simulink model "Basic_3ph"  (R2025a)
settings: Solver=VariableStepAuto  StartTime=0.0  StopTime=0.5  MaxStep=T_s  RelTol=1e-3
values from neighbouring files (symbols this model uses):
  Cdc = 500e-6    (= 0.0005)    [simulik_parameter_setter_inverter.m]
  f_e = 500    [simulik_parameter_setter_inverter.m]
  L_ph = 0.25e-3    (= 0.00025)    [simulik_parameter_setter_inverter.m]
  R_ph = 0.8e-3    (= 0.0008)    [ISCAD_Coupled_Model_3ph.m]
  T_s = 1/(20*f_sw)    [PowerElectronics_Analytical.m]    (also in simulik_parameter_setter_inverter.m = 2e-06)
  Td = 2e-6    (= 2e-06)    [PowerElectronics_Analytical.m]    (also in simulik_parameter_setter_inverter.m)
  Vdc = 48    [PowerElectronics_Analytical.m]    (also in simulik_parameter_setter_inverter.m)
undefined symbols (not defined in the file or in its folder): m
libraries: nesl_utility x14, fl_lib x9, ee_lib x6, eePwmGeneratorTwoLevel x1, spsRMSLib x1, spsThreePhaseSineGeneratorLib x1
settings Model: Creator=ossia  LastModifiedBy=ossia

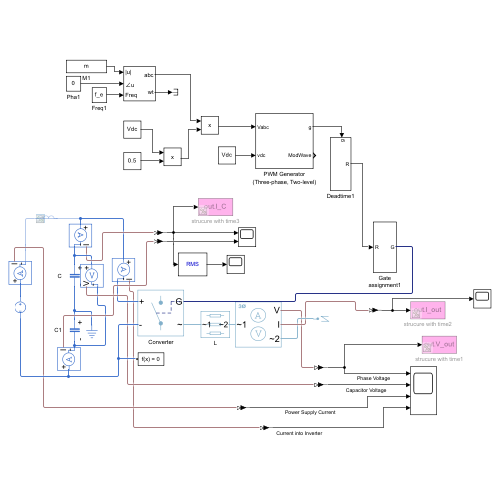
[thumbnail: Simulink's stored preview of the top-level diagram]
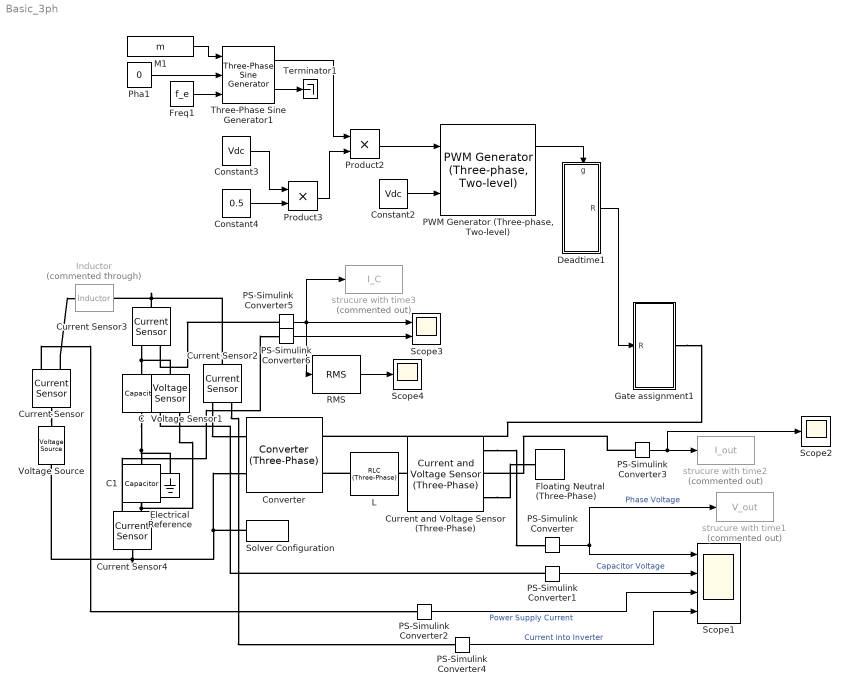
== system Basic_3ph ==
  C : fl_lib/Electrical/Electrical Elements/Capacitor  c=3*Cdc/2 uF  r=1e-4 Ohm  g=0 1/Ohm  i_specify=off  i_priority=High  i=0 A  i_nominal_specify=off  i_nominal_value=1  i_nominal_unit=A  v_specify=off  v_priority=None  v=Vdc/2 V  v_nominal_specify=off  v_nominal_value=1  v_nominal_unit=V  vc_specify=on  vc_priority=High  vc=Vdc/2 V  vc_nominal_specify=off  vc_nominal_value=1  vc_nominal_unit=V
  C1 : fl_lib/Electrical/Electrical Elements/Capacitor  c=3*Cdc/2 uF  r=1e-4 Ohm  g=0 1/Ohm  i_specify=off  i_priority=High  i=0 A  i_nominal_specify=off  i_nominal_value=1  i_nominal_unit=A  v_specify=off  v_priority=None  v=46 V  v_nominal_specify=off  v_nominal_value=1  v_nominal_unit=V  vc_specify=on  vc_priority=High  vc=Vdc/2 V  vc_nominal_specify=off  vc_nominal_value=1  vc_nominal_unit=V
  Constant2 : Constant  Value=Vdc
  Constant3 : Constant  Value=Vdc
  Constant4 : Constant  Value=0.5
  Converter : ee_lib/Semiconductors & Converters/Converters/Converter (Three-Phase)  port_option=ee.enum.threePhasePort.composite  fidelity_option=ee.enum.converters.fidelity.equivalent_pwm  device_type=ee.enum.converters.switchingdevice.mosfet  showThermalPort=false  K=0  Vth=0.5 V  Vgt=0.5 V  Vgt_off=0.1 V  Ih=1 A  Vf=0.6 V  Ron=0.002 Ohm  Rds=0.002 Ohm  Goff=1e-6 S  Eon_scalar=22.86e-3 J  Eoff_scalar=17.14e-3 J  Eoff_natural_commutation=10e-3 J  Voff=300 V  Iout_scalar=600 A  onCurrentMeasDelay=0 s  useCurrentFromPreviousCycle=false  useVoltageFromPreviousCycle=false  diode_param=2  diode_Vf=0.8 V  diode_Ron=0.001 Ohm  diode_Goff=1e-5 S  diode_C=5e-8 F  diode_iRM=-235 A  diode_iF=300 A  diode_idot=-50 A/us  diode_trr_param=1  diode_trr_factor=3  diode_trr=15 us  diode_Qrr=1.5e+3 s*uA  diode_rec_loss_model=ee.enum.diode.reverseRecoveryModel.fixed  diode_ErecVal=0 J  diode_scaleWithIandV=false  diode_ErecMat=zeros(2, 3) J  diode_TjrecVec=[298.15, 398.15] K  diode_IfrecVec=[.1, 1, 10] A  diode_IrecVal=10 A  diode_VrecVal=10 V  diode_tFilter=1 / 1000 / 100 s  thermal_network_parameterization=ee.enum.thermalNetworkTopology.external  Rth=[.08, .5] K/W  Rth_Cauer=[.08, .1, .5] K/W  Rth_Foster=[.08, .14, .22, .16] K/W  thermal_mass_parameterization=ee.enum.thermalNetwork.timeconstant  thermal_mass=[.01, .5] J/K  thermal_mass_Cauer=[.01, .1, .5] J/K  thermal_mass_Foster=[.001, .005, .05, .5] J/K  thermal_time_constant=[.001, .2] s  thermal_time_constant_Cauer=[.001, .1, .2] s  thermal_time_constant_Foster=[7e-05, .0007, .01, .08] s  thermal_mass_initial_temperatures=[25, 25] degC  thermal_mass_initial_temperatures_Cauer=[25, 25, 25] degC  junction_thermal_mass=0.01 J/K  Tvec_initial_Foster=[25, 25, 25, 25] degC  snubber_type=ee.enum.converters.snubber.exclude  Cs=1e-7 F  Rs=0.1 Ohm  Vce_loss=[0, 150, 300] V
  Current Sensor{,2..4} (4 alike) : fl_lib/Electrical/Electrical Sensors/Current Sensor
  Current and Voltage Sensor (Three-Phase) : ee_lib/Sensors & Transducers/Current and Voltage Sensor (Three-Phase)  vMeasurementType=ee.enum.vmeasurement.lg  outputUnit=ee.enum.unit.si  SRated=100e6 A*V  VRated=24e3 V  I_specify=off  I_priority=None  I=[0, 0, 0] A  I_nominal_specify=off  I_nominal_value=1  I_nominal_unit=A  V_specify=off  V_priority=None  V=[0, 0, 0] V  V_nominal_specify=off  V_nominal_value=1  V_nominal_unit=V
      settings: InternalSimscapePortConfiguration="{\"Bottom\":[],\"Left\":[{\"id\":\"N1\",\"label\":\"~1\",\"type\":\"foundation.electrical.three_phase\"}],\"Right\":[{\"id\":\"V_output\",\"label\":\"V\",\"type\":\"output\"},{\"id\":\"I_output\",\"label\":\"I\",\"type\":\"output\"},{\"id\":\"N2\",\"label\":\"~2\",\"type\":\"foundation.electrical.three_phase\"}],\"Top\":[]}"
  Deadtime1 : Subsystem
      settings: PortSchema="{\"entries\":[{\"content\":{\"sides\":[{\"content\":{\"connectorIds\":[\"Out1\"]},\"type\":\"ConnectorPlacement.EquallySpacedRectSide\",\"uuid\":\"80ef36b9-f465-4fcc-93a9-9d6eab044ae8\"},{\"content\":{\"side\":\"RIGHT\"},\"type\":\"ConnectorPlacement.EquallySpacedRectSide\",\"uuid\":\"10827d79-0026-467d-af8f-e653363972a6\"},{\"content\":{\"connectorIds\":[\"In1\"],\"side\":\"TOP\"},\"type\":\"ConnectorPlacement.EquallySpacedRectSide\",\"uuid\":\"d9163dac-283f-4784-a2ff-48ce53974a1a\"}]},\"type\":\"ConnectorPlacement.EquallySpacedConnector\",\"uuid\":\"7e643ad6-bdf3-49e0-97a6-0ece4f3a3f1f\"}],\"packageUris\":[\"http://schema.mathworks.com/mf0/Connector/R2020b\"],\"version\":\"1.0\"}"
  Electrical Reference : fl_lib/Electrical/Electrical Elements/Electrical Reference
  Floating Neutral (Three-Phase) : ee_lib/Connectors & References/Floating Neutral (Three-Phase)  G_parasitic=1e-12 1/Ohm
      settings: InternalSimscapePortConfiguration="{\"Bottom\":[],\"Left\":[{\"id\":\"N\",\"label\":\"~\",\"type\":\"foundation.electrical.three_phase\"}],\"Right\":[],\"Top\":[]}"
  Freq1 : Constant  Value=f_e
  Gate assignment1 : Subsystem
  Inductor : fl_lib/Electrical/Electrical Elements/Inductor  Commented=through  l=3*L_ph H  r=2e-3 Ohm  g=1e-9 1/Ohm  i_specify=off  i_priority=None  i=2 A  i_nominal_specify=off  i_nominal_value=1  i_nominal_unit=A  v_specify=off  v_priority=None  v=0 V  v_nominal_specify=off  v_nominal_value=1  v_nominal_unit=V  i_L_specify=off  i_L_priority=High  i_L=2 A  i_L_nominal_specify=off  i_L_nominal_value=1  i_L_nominal_unit=A
  L : ee_lib/Passive/RLC Assemblies/RLC (Three-Phase)  port_option=ee.enum.threePhasePort.composite  component_structure=4  R=R_ph Ohm  L=L_ph H  C=1e-6 F  R_parasitic=1e-6 Ohm  G_parasitic=1e-6 1/Ohm  IL_specify=on  IL_priority=High  IL=[ -14 7 7 ] A  IL_nominal_specify=off  IL_nominal_value=1  IL_nominal_unit=A  VC_specify=on  VC_priority=High  VC=[ 0 0 0 ] V  VC_nominal_specify=off  VC_nominal_value=1  VC_nominal_unit=V
      settings: InternalSimscapePortConfiguration="{\"Bottom\":[],\"Left\":[{\"id\":\"N1\",\"label\":\"~1\",\"type\":\"foundation.electrical.three_phase\"}],\"Right\":[{\"id\":\"N2\",\"label\":\"~2\",\"type\":\"foundation.electrical.three_phase\"}],\"Top\":[]}"
  M1 : Constant  Value=m
  PS-Simulink Converter{,1..6} (7 alike) : nesl_utility/PS-Simulink Converter  PhysicalDomain=network_engine_domain  SubClassName=ps_output  LeftPortType=input  RightPortType=output  PseudoPeriodic=off  Frequencies=[]  VectorFormat=inherit  Unit=inherit  AffineConversion=off
  "PWM Generator (Three-phase, Two-level)" : eePwmGeneratorTwoLevel/PWM Generator (Three-phase, Two-level)  PWMMode=Continuous PWM (CPWM)  CPWMMode=SPWM: sinusoidal PWM  DPWMMode=30 DPWM: 30 degree discontinuous PWM  fsw=f_sw  Ts=T_s
      settings: SamplingMode=Asymmetric
      settings: LibrarySourceBlock=|
      | ee_sl_lib/Pulse Width
      | Modulation/PWM Generator
      | (Three-phase, Two-level)
  Pha1 : Constant  Value=0
  Product2 : Product
  Product3 : Product
  RMS : spsRMSLib/RMS  TrueRMS=on  Freq=25  RMSInit=0  Ts=T_s
  Scope1 : Scope  NumInputPorts=4
      settings: ActiveDisplayYMinimum=-29.00001636217473  ActiveDisplayYMaximum=21.000035118664378
  Scope2 : Scope
      settings: ActiveDisplayYMinimum=-1023.5079890337755  ActiveDisplayYMaximum=992.075721007424  DataLoggingVariableName=ScopeData2
  Scope3 : Scope  NumInputPorts=2
      settings: ActiveDisplayYMinimum=-298.34389890666739  ActiveDisplayYMaximum=287.62683048751734  DataLoggingVariableName=ScopeData3
  Scope4 : Scope
      settings: ActiveDisplayYMinimum=-372.34194  ActiveDisplayYMaximum=490.06934
  Solver Configuration : nesl_utility/Solver Configuration  PhysicalDomain=network_engine_domain  SubClassName=solver  LeftPortType=input  RightPortType=generic  Tones=[]  Harmonics=[]  SimulateNoise=off  Profile=off  UseLocalSampling=off  EnableSwitchedLinearOptims=on  FrequencyDomain=off  UseCCode=off  RelTol=0.001  AbsTol=1e-06  MinStep=1e-09  ToWorkspace=off  RevertToSquareIcSolve=off  NumHomotopyIterations=100  PhasorMode=off  PhasorModeNumHarmonics=1  ConsistencySolver=NEWTON_FTOL  IndexReductionMethod=DerivativeReplacement  DoDC=off  ResidualTolerance=1e-09  ConsistencyTolSource=GLOBAL  ConsistencyAbsTol=0.001  ConsistencyRelTol=0.001  ConsistencyTolFactor=0.001  UseLocalSolver=off  LocalSolverChoice=NE_BACKWARD_EULER_ADVANCER  ResolveIndetEquations=on  FunctionEvalNumThread=1  LocalSolverSampleTime=1e-5  DoFixedCost=off  MaxNonlinIter=5  MaxModeIter=2  ComputeImpulses=off  ImpulseIterations=2  LinearAlgebra=Sparse  LinearAlgebraNumThread=0  EquationFormulation=NE_TIME_EF  DelaysMemoryBudget=1024  AutomaticFiltering=on  FilteringTimeConstant=0.001  PartitionStorageMethod=AS_NEEDED  PartitionMemoryBudget=1024  PartitionMethod=FAST  MultibodyUseLocalSolver=off  MultibodyLocalSolverChoice=ODE1  MultibodyLocalSolverSampleTime=0.001
  Terminator1 : Terminator
  Three-Phase Sine Generator1 : spsThreePhaseSineGeneratorLib/Three-Phase Sine Generator  Ts=T_s
      settings: LibrarySourceBlock=|
      | sps_lib/Sources/Signal Generator Sources/Three-Phase
      | Sine Generator
  Voltage Sensor1 : fl_lib/Electrical/Electrical Sensors/Voltage Sensor
  Voltage Source : ee_lib/Sources/Voltage Source  dc_voltage=Vdc V  ac_voltage=0 V  ac_shift=0 rad  ac_frequency=0 Hz  noise_mode=ee.enum.sources.noise.Disabled  PSD=0 V^2/Hz  sample_time=1e-3 s  repeatability=ee.enum.sources.repeatability.NotRepeatable  user_seed=0  auto_seed=3890346746  i_specify=off  i_priority=None  i=0 A  i_nominal_specify=off  i_nominal_value=1  i_nominal_unit=A  v_specify=off  v_priority=None  v=0 V  v_nominal_specify=off  v_nominal_value=1  v_nominal_unit=V
  strucure with time1 : ToWorkspace  Commented=on  VariableName=V_out  SaveFormat=Structure With Time  SampleTime=T_s
  strucure with time2 : ToWorkspace  Commented=on  VariableName=I_out  SaveFormat=Structure With Time  SampleTime=T_s
  strucure with time3 : ToWorkspace  Commented=on  VariableName=I_C  SaveFormat=Structure With Time  SampleTime=T_s
  wires:
  PS-Simulink Converter/1 -> strucure with time1/1, Scope1/1  "Phase Voltage"
  Constant4/1 -> Product3/2
  Three-Phase Sine Generator1/1 -> Product2/1
  Freq1/1 -> Three-Phase Sine Generator1/3
  PS-Simulink Converter1/1 -> Scope1/2  "Capacitor Voltage"
  Deadtime1/1(R) -> Gate assignment1/1(R)
  Pha1/1 -> Three-Phase Sine Generator1/2
  PS-Simulink Converter6/1 -> Scope3/2
  Three-Phase Sine Generator1/2 -> Terminator1/1
  Constant2/1 -> "PWM Generator (Three-phase, Two-level)"/2
  Product2/1 -> "PWM Generator (Three-phase, Two-level)"/1
  "PWM Generator (Three-phase, Two-level)"/1 -> Deadtime1/1(g)
  PS-Simulink Converter2/1 -> Scope1/3  "Power Supply Current"
  PS-Simulink Converter3/1 -> Scope2/1, strucure with time2/1
  Product3/1 -> Product2/2
  PS-Simulink Converter5/1 -> strucure with time3/1, RMS/1, Scope3/1
  RMS/1 -> Scope4/1
  Constant3/1 -> Product3/1
  PS-Simulink Converter4/1 -> Scope1/4  "Current into Inverter"
  M1/1 -> Three-Phase Sine Generator1/1
  connections:
  Converter/RConn2 -- Solver Configuration/RConn1 -- Current Sensor4/LConn1 -- Voltage Source/RConn1
  C1/LConn1 -- C/RConn1 -- Electrical Reference/LConn1
  C/LConn1 -- Voltage Sensor1/LConn1 -- Current Sensor3/RConn2
  Current Sensor3/LConn1 -- Current Sensor2/LConn1 -- Inductor/RConn1
  PS-Simulink Converter5/LConn1 -- Current Sensor3/RConn1
  Current Sensor/RConn2 -- Inductor/LConn1
  PS-Simulink Converter1/LConn1 -- Voltage Sensor1/RConn1
  Current Sensor/RConn1 -- PS-Simulink Converter2/LConn1
  PS-Simulink Converter3/LConn1 -- Current and Voltage Sensor (Three-Phase)/RConn2
  Current Sensor4/RConn1 -- PS-Simulink Converter6/LConn1
  Current Sensor2/RConn1 -- PS-Simulink Converter4/LConn1
  Gate assignment1/RConn1 -- Converter/LConn1
  Current Sensor4/RConn2 -- Voltage Sensor1/RConn2 -- C1/RConn1
  Current Sensor2/RConn2 -- Converter/RConn1
  Current Sensor/LConn1 -- Voltage Source/LConn1
  Current and Voltage Sensor (Three-Phase)/RConn1 -- PS-Simulink Converter/LConn1
  L/LConn1 -- Converter/LConn2
  Current and Voltage Sensor (Three-Phase)/LConn1 -- L/RConn1
  Current and Voltage Sensor (Three-Phase)/RConn3 -- Floating Neutral (Three-Phase)/LConn1

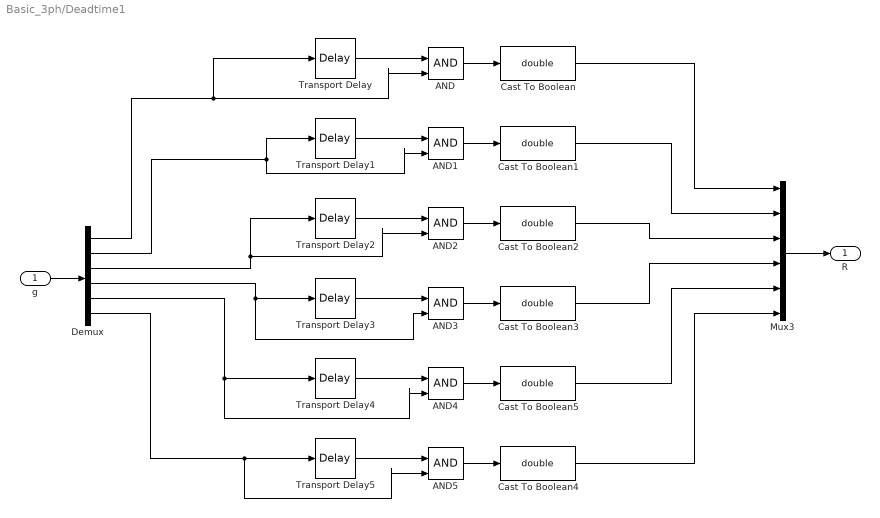
== system Basic_3ph/Deadtime1 ==
  g : Inport
  AND{,1..5} (6 alike) : Logic  IconShape=distinctive  AllPortsSameDT=off  OutDataTypeStr=boolean
  Cast To Boolean{,1..5} (6 alike) : DataTypeConversion  OutDataTypeStr=double  SaturateOnIntegerOverflow=off  RndMeth=Floor
  Demux : Demux  Outputs=6
  Mux3 : Mux  Inputs=6
  Transport Delay{,1..5} (6 alike) : TransportDelay  DelayTime=Td
  R : Outport
  wires:
  g/1 -> Demux/1
  Transport Delay/1 -> AND/1
  Demux/1 -> Transport Delay/1, AND/2
  AND/1 -> Cast To Boolean/1
  Demux/2 -> Transport Delay1/1, AND1/2
  Transport Delay1/1 -> AND1/1
  Transport Delay2/1 -> AND2/1
  AND2/1 -> Cast To Boolean2/1
  Demux/3 -> Transport Delay2/1, AND2/2
  Demux/4 -> AND3/2, Transport Delay3/1
  Transport Delay3/1 -> AND3/1
  Demux/5 -> AND4/2, Transport Delay4/1
  Transport Delay4/1 -> AND4/1
  AND4/1 -> Cast To Boolean5/1
  Demux/6 -> AND5/2, Transport Delay5/1
  Transport Delay5/1 -> AND5/1
  AND1/1 -> Cast To Boolean1/1
  AND3/1 -> Cast To Boolean3/1
  AND5/1 -> Cast To Boolean4/1
  Cast To Boolean/1 -> Mux3/1
  Cast To Boolean1/1 -> Mux3/2
  Cast To Boolean2/1 -> Mux3/3
  Cast To Boolean3/1 -> Mux3/4
  Cast To Boolean5/1 -> Mux3/5
  Cast To Boolean4/1 -> Mux3/6
  Mux3/1 -> R/1

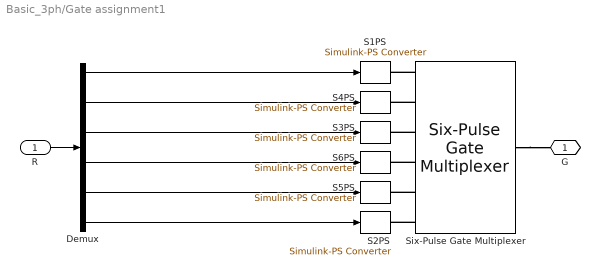
== system Basic_3ph/Gate assignment1 ==
  R : Inport
  Demux : Demux  Outputs=6
  S1PS : nesl_utility/Simulink-PS Converter  PhysicalDomain=network_engine_domain  SubClassName=ps_input  LeftPortType=input  RightPortType=output  PseudoPeriodic=off  Frequencies=[]  NoiseDistribution=none  NoiseParameters=[]  Unit=1  AffineConversion=off  FilteringAndDerivatives=zero  SimscapeFilterOrder=1  InputFilterTimeConstant=.001  UdotUserProvided=1
  S2PS : nesl_utility/Simulink-PS Converter  PhysicalDomain=network_engine_domain  SubClassName=ps_input  LeftPortType=input  RightPortType=output  PseudoPeriodic=off  Frequencies=[]  NoiseDistribution=none  NoiseParameters=[]  Unit=1  AffineConversion=off  FilteringAndDerivatives=zero  SimscapeFilterOrder=1  InputFilterTimeConstant=.001  UdotUserProvided=[]
  S3PS : nesl_utility/Simulink-PS Converter  PhysicalDomain=network_engine_domain  SubClassName=ps_input  LeftPortType=input  RightPortType=output  PseudoPeriodic=off  Frequencies=[]  NoiseDistribution=none  NoiseParameters=[]  Unit=1  AffineConversion=off  FilteringAndDerivatives=zero  SimscapeFilterOrder=1  InputFilterTimeConstant=.001  UdotUserProvided=[]
  S4PS : nesl_utility/Simulink-PS Converter  PhysicalDomain=network_engine_domain  SubClassName=ps_input  LeftPortType=input  RightPortType=output  PseudoPeriodic=off  Frequencies=[]  NoiseDistribution=none  NoiseParameters=[]  Unit=1  AffineConversion=off  FilteringAndDerivatives=zero  SimscapeFilterOrder=1  InputFilterTimeConstant=.001  UdotUserProvided=[]
  S5PS : nesl_utility/Simulink-PS Converter  PhysicalDomain=network_engine_domain  SubClassName=ps_input  LeftPortType=input  RightPortType=output  PseudoPeriodic=off  Frequencies=[]  NoiseDistribution=none  NoiseParameters=[]  Unit=1  AffineConversion=off  FilteringAndDerivatives=zero  SimscapeFilterOrder=1  InputFilterTimeConstant=.001  UdotUserProvided=[]
  S6PS : nesl_utility/Simulink-PS Converter  PhysicalDomain=network_engine_domain  SubClassName=ps_input  LeftPortType=input  RightPortType=output  PseudoPeriodic=off  Frequencies=[]  NoiseDistribution=none  NoiseParameters=[]  Unit=1  AffineConversion=off  FilteringAndDerivatives=zero  SimscapeFilterOrder=1  InputFilterTimeConstant=.001  UdotUserProvided=[]
  Six-Pulse Gate Multiplexer : ee_lib/Semiconductors & Converters/Converters/Six-Pulse Gate Multiplexer  port_option=ee.enum.controlport.ps
  G : PMIOPort  Side=Right
  wires:
  R/1 -> Demux/1
  Demux/1 -> S1PS/1
  Demux/2 -> S4PS/1
  Demux/3 -> S3PS/1
  Demux/4 -> S6PS/1
  Demux/5 -> S5PS/1
  Demux/6 -> S2PS/1
  connections:
  Six-Pulse Gate Multiplexer/LConn1 -- S1PS/RConn1
  Six-Pulse Gate Multiplexer/LConn2 -- S4PS/RConn1
  Six-Pulse Gate Multiplexer/RConn1 -- G/RConn1
  Six-Pulse Gate Multiplexer/LConn3 -- S3PS/RConn1
  Six-Pulse Gate Multiplexer/LConn6 -- S2PS/RConn1
  Six-Pulse Gate Multiplexer/LConn5 -- S5PS/RConn1
  Six-Pulse Gate Multiplexer/LConn4 -- S6PS/RConn1
